simulink subsystem "ControlSystem"  (R2023b)
settings: Solver=VariableStepAuto  StartTime=0.0  StopTime=10.0  RelTol=1e-3
undefined symbols (not defined in the file): Acl, Acld, Bcl, Bcld, Ccl, Ccld, Dcl, Dcld, dt, EOL_Vehicle_Speed, Kgain, Ksgain
settings Model: Creator=konur  LastModifiedBy=konur

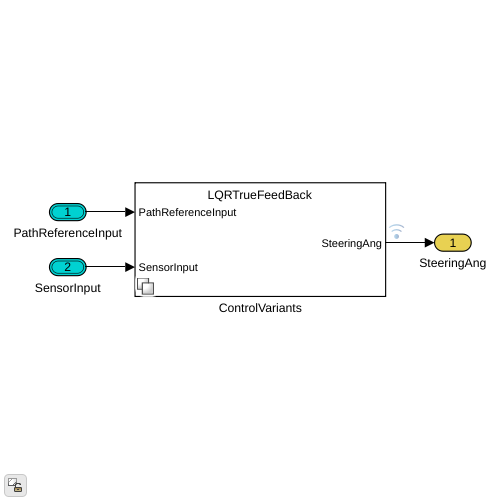
[thumbnail: Simulink's stored preview of the top-level diagram]
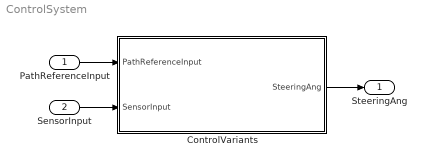
== system ControlSystem ==
  PathReferenceInput : Inport  OutDataTypeStr=Bus: PathManagerOut
  SensorInput : Inport  Port=2  OutDataTypeStr=Bus: VehicleModelBus
  ControlVariants : Subsystem  Variant=on
  SteeringAng : Outport  OutDataTypeStr=double
  wires:
  SensorInput/1 -> ControlVariants/2(SensorInput)
  ControlVariants/1(SteeringAng) -> SteeringAng/1
  PathReferenceInput/1 -> ControlVariants/1(PathReferenceInput)

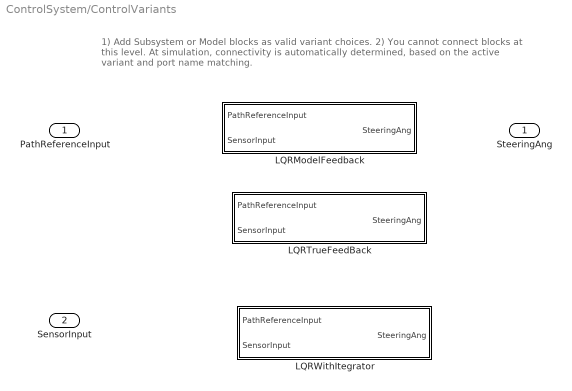
== system ControlSystem/ControlVariants ==
  note: 1) Add Subsystem or Model blocks as valid variant choices.
      | 2) You cannot connect blocks at this level. At simulation, connectivity is automatically
      | determined, based on the active variant and port name matching.
  PathReferenceInput : Inport  OutDataTypeStr=Bus: PathManagerOut
  SensorInput : Inport  Port=2  OutDataTypeStr=Bus: VehicleModelBus
  LQRModelFeedback : Subsystem  VariantControl=ControlVariant==1
  LQRTrueFeedBack : Subsystem  VariantControl=ControlVariant==2
  LQRWithItegrator : Subsystem  VariantControl=ControlVariant==3
  SteeringAng : Outport

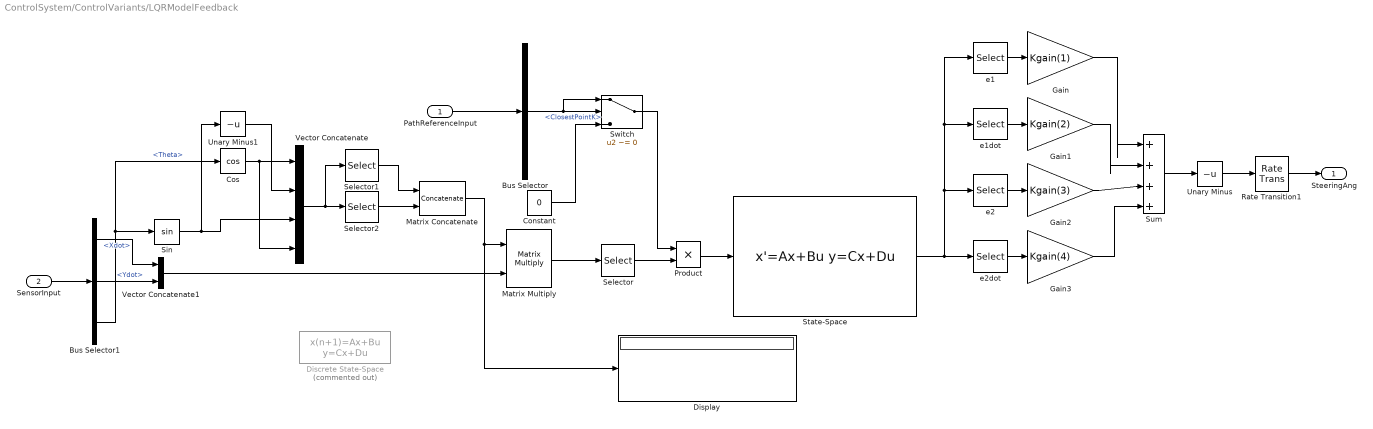
== system ControlSystem/ControlVariants/LQRModelFeedback ==
  PathReferenceInput : Inport  OutDataTypeStr=Bus: PathManagerOut
  SensorInput : Inport  Port=2  OutDataTypeStr=Bus: VehicleModelBus
  Bus Selector : BusSelector  OutputSignals=ClosestPointK
  Bus Selector1 : BusSelector  OutputSignals=Xdot,Ydot,Theta
  Constant : Constant  Value=0
  Cos : Trigonometry  Operator=cos
  Discrete State-Space : DiscreteStateSpace  Commented=on  A=Acld  B=Bcld  C=Ccld  D=Dcld  SampleTime=dt
  Display : Display
  Gain : Gain  Gain=Kgain(1)  OutDataTypeStr=double
  Gain1 : Gain  Gain=Kgain(2)
  Gain2 : Gain  Gain=Kgain(3)
  Gain3 : Gain  Gain=Kgain(4)
  Matrix Concatenate : Concatenate  Mode=Multidimensional array  ConcatenateDimension=2
  Matrix Multiply : Product  Multiplication=Matrix(*)
  Product : Product
  Rate Transition1 : RateTransition
  Selector : Selector  InputPortWidth=2  IndexOptions=Index vector (dialog)  Indices=[1]  OutputSizes=1
  Selector1 : Selector  InputPortWidth=4  IndexOptions=Index vector (dialog)  Indices=[1 2]  OutputSizes=1
  Selector2 : Selector  InputPortWidth=4  IndexOptions=Index vector (dialog)  Indices=[3 4]  OutputSizes=1
  Sin : Trigonometry
  State-Space : StateSpace  A=Acl  B=Bcl  C=Ccl  D=Dcl  InitialCondition=0
  Sum : Sum  Inputs=|++++  OutDataTypeStr=double
  Switch : Switch  Criteria=u2 ~= 0  SaturateOnIntegerOverflow=off  InputSameDT=off
  Unary Minus : UnaryMinus
  Unary Minus1 : UnaryMinus
  Vector Concatenate : Concatenate  NumInputs=4
  Vector Concatenate1 : Concatenate
  e1 : Selector  InputPortWidth=4  IndexOptions=Index vector (dialog)  Indices=1  OutputSizes=1
  e1dot : Selector  InputPortWidth=4  IndexOptions=Index vector (dialog)  Indices=2  OutputSizes=1
  e2 : Selector  InputPortWidth=4  IndexOptions=Index vector (dialog)  Indices=3  OutputSizes=1
  e2dot : Selector  InputPortWidth=4  IndexOptions=Index vector (dialog)  Indices=4  OutputSizes=1
  SteeringAng : Outport  OutDataTypeStr=double
  wires:
  Gain3/1 -> Sum/4
  Vector Concatenate1/1 -> Matrix Multiply/2
  Gain2/1 -> Sum/3
  Gain1/1 -> Sum/2
  Gain/1 -> Sum/1
  e2dot/1 -> Gain3/1
  e1/1 -> Gain/1
  Product/1 -> State-Space/1
  Selector/1 -> Product/2
  Sum/1 -> Unary Minus/1
  Matrix Multiply/1 -> Selector/1
  Bus Selector/1 -> Switch/2, Switch/1  "<ClosestPointK>"
  Sin/1 -> Vector Concatenate/3, Unary Minus1/1
  Bus Selector1/1 -> Vector Concatenate1/1  "<Xdot>"
  Selector2/1 -> Matrix Concatenate/2
  Selector1/1 -> Matrix Concatenate/1
  SensorInput/1 -> Bus Selector1/1
  PathReferenceInput/1 -> Bus Selector/1
  Bus Selector1/2 -> Vector Concatenate1/2  "<Ydot>"
  Bus Selector1/3 -> Cos/1, Sin/1  "<Theta>"
  Switch/1 -> Product/1
  Unary Minus1/1 -> Vector Concatenate/2
  Cos/1 -> Vector Concatenate/1, Vector Concatenate/4
  e1dot/1 -> Gain1/1
  State-Space/1 -> e2dot/1, e2/1, e1dot/1, e1/1
  Vector Concatenate/1 -> Selector1/1, Selector2/1
  Constant/1 -> Switch/3
  Matrix Concatenate/1 -> Matrix Multiply/1, Display/1
  e2/1 -> Gain2/1
  Unary Minus/1 -> Rate Transition1/1
  Rate Transition1/1 -> SteeringAng/1

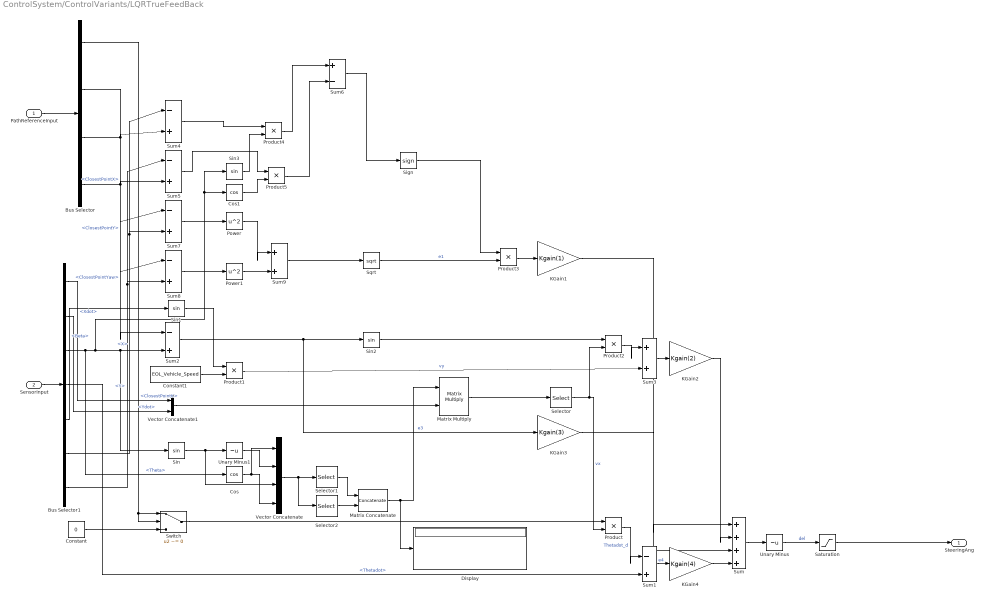
== system ControlSystem/ControlVariants/LQRTrueFeedBack ==
  PathReferenceInput : Inport  OutDataTypeStr=Bus: PathManagerOut
  SensorInput : Inport  Port=2  OutDataTypeStr=Bus: VehicleModelBus
  Bus Selector : BusSelector  OutputSignals=ClosestPointK,ClosestPointYaw,ClosestPointX,ClosestPointY
  Bus Selector1 : BusSelector  OutputSignals=Xdot,Ydot,Theta,Thetadot,Beta,X,Y
  Constant : Constant  Value=0
  Constant1 : Constant  Value=EOL_Vehicle_Speed  OutDataTypeStr=double
  Cos : Trigonometry  Operator=cos  OutputSignalType=real
  Cos1 : Trigonometry  Operator=cos
  Display : Display
  KGain1 : Gain  Gain=Kgain(1)  OutDataTypeStr=double
  KGain2 : Gain  Gain=Kgain(2)
  KGain3 : Gain  Gain=Kgain(3)
  KGain4 : Gain  Gain=Kgain(4)
  Matrix Concatenate : Concatenate  Mode=Multidimensional array  ConcatenateDimension=2
  Matrix Multiply : Product  Multiplication=Matrix(*)
  Power : Math  Operator=square  OutDataTypeStr=double
  Power1 : Math  Operator=square  OutDataTypeStr=double
  Product{,1,3..5} (5 alike) : Product
  Product2 : Product  OutDataTypeStr=double
  Saturation : Saturate  UpperLimit=pi/5  LowerLimit=-pi/5
  Selector : Selector  InputPortWidth=2  IndexOptions=Index vector (dialog)  Indices=[1]  OutputSizes=1
  Selector1 : Selector  InputPortWidth=4  IndexOptions=Index vector (dialog)  Indices=[1 2]  OutputSizes=1
  Selector2 : Selector  InputPortWidth=4  IndexOptions=Index vector (dialog)  Indices=[3 4]  OutputSizes=1
  Sign : Signum
  Sin : Trigonometry  OutputSignalType=real
  Sin1 : Trigonometry
  Sin2 : Trigonometry  OutputSignalType=real
  Sin3 : Trigonometry
  Sqrt : Sqrt
  Sum : Sum  Inputs=|++++  OutDataTypeStr=double
  Sum1 : Sum  Inputs=|-+
  Sum2 : Sum  Inputs=|-+
  Sum3 : Sum  Inputs=|++  OutDataTypeStr=double
  Sum{4..5,7..8} (4 alike) : Sum  Inputs=|-+  OutDataTypeStr=double
  Sum6 : Sum  Inputs=|+-  OutDataTypeStr=double
  Sum9 : Sum  Inputs=|++  OutDataTypeStr=double
  Switch : Switch  Criteria=u2 ~= 0  SaturateOnIntegerOverflow=off  InputSameDT=off
  Unary Minus : UnaryMinus
  Unary Minus1 : UnaryMinus
  Vector Concatenate : Concatenate  NumInputs=4
  Vector Concatenate1 : Concatenate
  SteeringAng : Outport  OutDataTypeStr=double
  wires:
  Product5/1 -> Sum6/2
  Product4/1 -> Sum6/1
  Power1/1 -> Sum9/2
  Power/1 -> Sum9/1
  Bus Selector/3 -> Sum7/1, Sum4/2  "<ClosestPointX>"
  Vector Concatenate1/1 -> Matrix Multiply/2
  Bus Selector1/3 -> Cos/1, Sin/1, Sum2/2, Sin3/1, Cos1/1  "<Theta>"
  KGain1/1 -> Sum/1
  Cos1/1 -> Product5/2
  Sum2/1 -> KGain3/1, Sin2/1  "e3"
  Sum8/1 -> Power1/1
  Sum7/1 -> Power/1
  KGain4/1 -> Sum/4
  Sum5/1 -> Product5/1
  Sin/1 -> Vector Concatenate/3, Unary Minus1/1
  Selector/1 -> Product2/2, Product/2  "vx"
  Sin3/1 -> Product4/2
  Bus Selector/2 -> Sum2/1  "<ClosestPointYaw>"
  Vector Concatenate/1 -> Selector2/1, Selector1/1
  Switch/1 -> Product/1
  Bus Selector1/6 -> Sum4/1, Sum7/2  "<X>"
  Constant/1 -> Switch/3
  PathReferenceInput/1 -> Bus Selector/1
  SensorInput/1 -> Bus Selector1/1
  Bus Selector/1 -> Switch/2, Switch/1  "<ClosestPointK>"
  Bus Selector1/1 -> Vector Concatenate1/1  "<Xdot>"
  Bus Selector1/7 -> Sum5/1, Sum8/2  "<Y>"
  Sum4/1 -> Product4/1
  Product/1 -> Sum1/1  "Thetadot_d"
  Bus Selector1/5 -> Sin1/1  "<Beta>"
  Bus Selector1/4 -> Sum1/2  "<Thetadot>"
  Sin1/1 -> Product1/1
  Bus Selector/4 -> Sum8/1, Sum5/2  "<ClosestPointY>"
  Product1/1 -> Sum3/2  "vy"
  Constant1/1 -> Product1/2
  Bus Selector1/2 -> Vector Concatenate1/2  "<Ydot>"
  Unary Minus1/1 -> Vector Concatenate/2
  Cos/1 -> Vector Concatenate/4, Vector Concatenate/1
  Sum1/1 -> KGain4/1  "e4"
  Sum6/1 -> Sign/1
  Selector2/1 -> Matrix Concatenate/2
  Sum9/1 -> Sqrt/1
  Selector1/1 -> Matrix Concatenate/1
  Sign/1 -> Product3/1
  Sqrt/1 -> Product3/2  "e1"
  Sin2/1 -> Product2/1
  Matrix Concatenate/1 -> Display/1, Matrix Multiply/1
  Product3/1 -> KGain1/1
  Matrix Multiply/1 -> Selector/1
  Sum3/1 -> KGain2/1
  Unary Minus/1 -> Saturation/1  "del"
  KGain3/1 -> Sum/3
  Product2/1 -> Sum3/1
  KGain2/1 -> Sum/2
  Sum/1 -> Unary Minus/1
  Saturation/1 -> SteeringAng/1

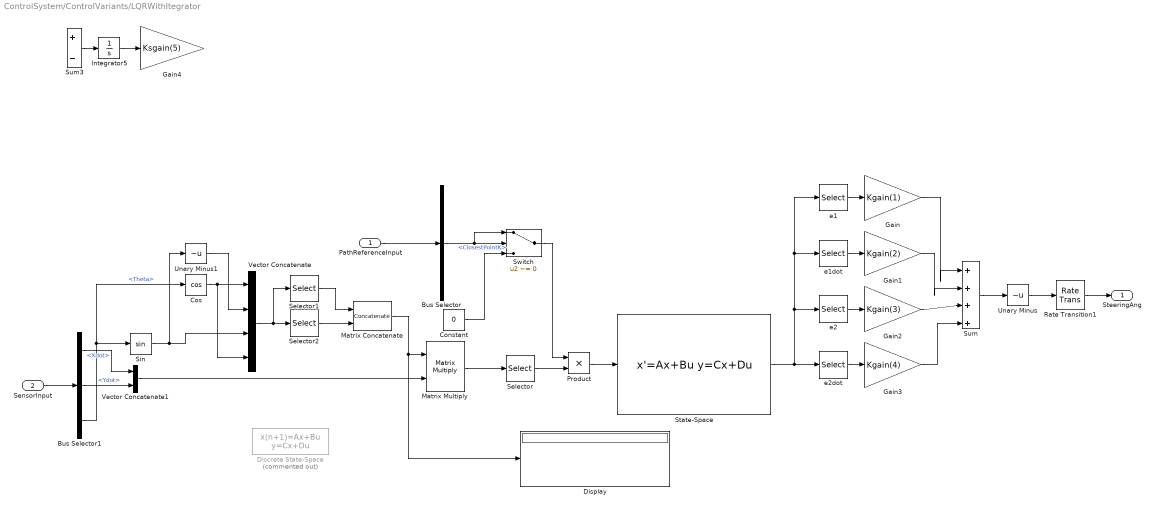
== system ControlSystem/ControlVariants/LQRWithItegrator ==
  PathReferenceInput : Inport  OutDataTypeStr=Bus: PathManagerOut
  SensorInput : Inport  Port=2  OutDataTypeStr=Bus: VehicleModelBus
  Bus Selector : BusSelector  OutputSignals=ClosestPointK
  Bus Selector1 : BusSelector  OutputSignals=Xdot,Ydot,Theta
  Constant : Constant  Value=0
  Cos : Trigonometry  Operator=cos
  Discrete State-Space : DiscreteStateSpace  Commented=on  A=Acld  B=Bcld  C=Ccld  D=Dcld  SampleTime=dt
  Display : Display
  Gain : Gain  Gain=Kgain(1)  OutDataTypeStr=double
  Gain1 : Gain  Gain=Kgain(2)
  Gain2 : Gain  Gain=Kgain(3)
  Gain3 : Gain  Gain=Kgain(4)
  Gain4 : Gain  Gain=Ksgain(5)  OutDataTypeStr=double
  Integrator5 : Integrator
  Matrix Concatenate : Concatenate  Mode=Multidimensional array  ConcatenateDimension=2
  Matrix Multiply : Product  Multiplication=Matrix(*)
  Product : Product
  Rate Transition1 : RateTransition
  Selector : Selector  InputPortWidth=2  IndexOptions=Index vector (dialog)  Indices=[1]  OutputSizes=1
  Selector1 : Selector  InputPortWidth=4  IndexOptions=Index vector (dialog)  Indices=[1 2]  OutputSizes=1
  Selector2 : Selector  InputPortWidth=4  IndexOptions=Index vector (dialog)  Indices=[3 4]  OutputSizes=1
  Sin : Trigonometry
  State-Space : StateSpace  A=Acl  B=Bcl  C=Ccl  D=Dcl  InitialCondition=0
  Sum : Sum  Inputs=|++++  OutDataTypeStr=double
  Sum3 : Sum  Inputs=|+-  OutDataTypeStr=double
  Switch : Switch  Criteria=u2 ~= 0  SaturateOnIntegerOverflow=off  InputSameDT=off
  Unary Minus : UnaryMinus
  Unary Minus1 : UnaryMinus
  Vector Concatenate : Concatenate  NumInputs=4
  Vector Concatenate1 : Concatenate
  e1 : Selector  InputPortWidth=4  IndexOptions=Index vector (dialog)  Indices=1  OutputSizes=1
  e1dot : Selector  InputPortWidth=4  IndexOptions=Index vector (dialog)  Indices=2  OutputSizes=1
  e2 : Selector  InputPortWidth=4  IndexOptions=Index vector (dialog)  Indices=3  OutputSizes=1
  e2dot : Selector  InputPortWidth=4  IndexOptions=Index vector (dialog)  Indices=4  OutputSizes=1
  SteeringAng : Outport  OutDataTypeStr=double
  wires:
  Gain3/1 -> Sum/4
  Sum/1 -> Unary Minus/1
  Gain2/1 -> Sum/3
  Cos/1 -> Vector Concatenate/1, Vector Concatenate/4
  Gain/1 -> Sum/1
  State-Space/1 -> e2dot/1, e2/1, e1dot/1, e1/1
  Matrix Concatenate/1 -> Matrix Multiply/1, Display/1
  e2dot/1 -> Gain3/1
  SensorInput/1 -> Bus Selector1/1
  Gain1/1 -> Sum/2
  Selector/1 -> Product/2
  Vector Concatenate1/1 -> Matrix Multiply/2
  Selector1/1 -> Matrix Concatenate/1
  e1/1 -> Gain/1
  e2/1 -> Gain2/1
  Product/1 -> State-Space/1
  Switch/1 -> Product/1
  Bus Selector1/2 -> Vector Concatenate1/2  "<Ydot>"
  PathReferenceInput/1 -> Bus Selector/1
  Bus Selector1/3 -> Cos/1, Sin/1  "<Theta>"
  Constant/1 -> Switch/3
  e1dot/1 -> Gain1/1
  Bus Selector1/1 -> Vector Concatenate1/1  "<Xdot>"
  Unary Minus/1 -> Rate Transition1/1
  Selector2/1 -> Matrix Concatenate/2
  Sin/1 -> Vector Concatenate/3, Unary Minus1/1
  Bus Selector/1 -> Switch/2, Switch/1  "<ClosestPointK>"
  Matrix Multiply/1 -> Selector/1
  Unary Minus1/1 -> Vector Concatenate/2
  Rate Transition1/1 -> SteeringAng/1
  Vector Concatenate/1 -> Selector1/1, Selector2/1
  Integrator5/1 -> Gain4/1
  Sum3/1 -> Integrator5/1
